simulink model "ebenes_quellenfreies_Windfeld"  (R2020b)
settings: Solver=VariableStepAuto  StartTime=0.0  StopTime=100  RelTol=1e-3
settings Model: Creator=Dogukan  LastModifiedBy=Dogukan

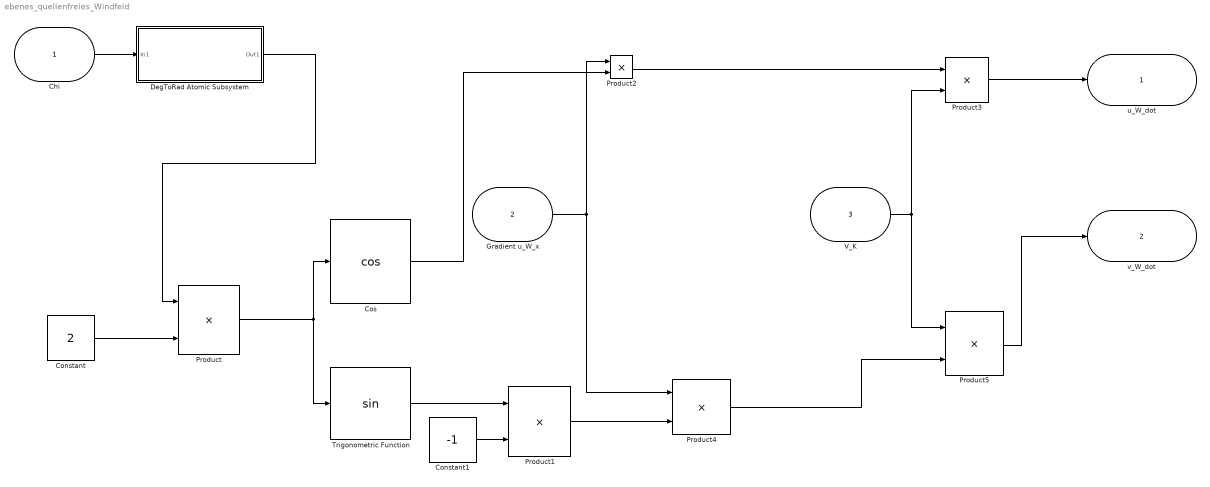
== system ebenes_quellenfreies_Windfeld ==
  Chi : Inport
  Gradient u_W_x : Inport  Port=2
  V_K : Inport  Port=3
  Constant : Constant  Value=2
  Constant1 : Constant  Value=-1
  Cos : Trigonometry  Operator=cos
  DegToRad Atomic Subsystem : Subsystem  TreatAsAtomicUnit=on
  Product{,1..5} (6 alike) : Product
  Trigonometric Function : Trigonometry
  u_W_dot : Outport
  v_W_dot : Outport  Port=2
  wires:
  Constant/1 -> Product/2
  Product/1 -> Trigonometric Function/1, Cos/1
  Constant1/1 -> Product1/2
  Trigonometric Function/1 -> Product1/1
  Gradient u_W_x/1 -> Product4/1, Product2/1
  Cos/1 -> Product2/2
  Product2/1 -> Product3/1
  V_K/1 -> Product3/2, Product5/1
  Product3/1 -> u_W_dot/1
  Product1/1 -> Product4/2
  Product4/1 -> Product5/2
  Product5/1 -> v_W_dot/1
  DegToRad Atomic Subsystem/1(Out1) -> Product/1
  Chi/1 -> DegToRad Atomic Subsystem/1(In1)

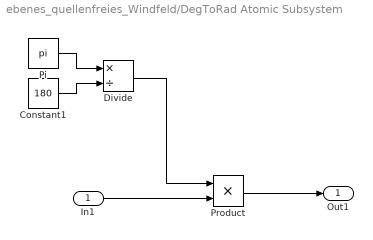
== system ebenes_quellenfreies_Windfeld/DegToRad Atomic Subsystem ==
  In1 : Inport
  Constant1 : Constant  Value=180
  Divide : Product  Inputs=*/
  Pi : Constant  Value=pi  OutDataTypeStr=Inherit: Inherit via back propagation
  Product : Product
  Out1 : Outport
  wires:
  Pi/1 -> Divide/1
  Constant1/1 -> Divide/2
  Divide/1 -> Product/1
  In1/1 -> Product/2
  Product/1 -> Out1/1
